simulink model "FixedWingPathDynamics"  (R2021b)
settings: Solver=VariableStepAuto  StartTime=0.0  StopTime=210  RelTol=1e-3
InitFcn:
  | FidelityStage = 2;
model workspace (MAT data in the model file):
  airspeedVal = 12.0293777094
  headingAngles : timeseries (value not decoded)
  lastWaypointInstance = [-187.583573788; -374.036820677; -81.0768]
  lookaheadPoint : timeseries (value not decoded)
  waypointData = [-39.8122089943 -39.8116872817 -39.8111647517 -39.8106414064 -39.8101172475 -39.809592277 -39.8090664968 -39.8085399087 -39.8080125146 -39.8074843164 -39.80695542 -39.8064258792 ... (1797 elements, 599x3)]
undefined symbols (not defined in the file): aircraftTmax, initialThrottle, midFidelityUAV, trimT
libraries: aerolibconvert2 x1, uavalgslib x1
(part 2 of 2)

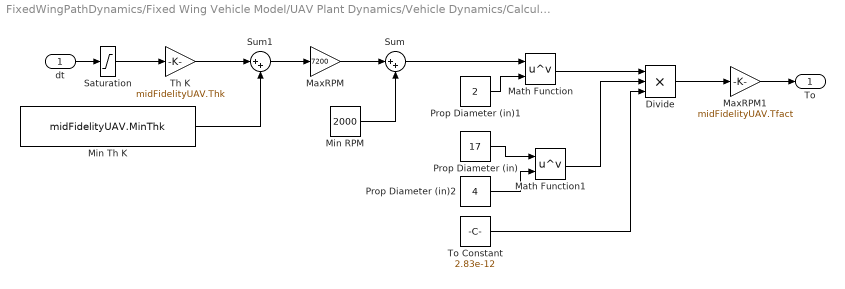
== system FixedWingPathDynamics/Fixed Wing Vehicle Model/UAV Plant Dynamics/Vehicle Dynamics/Calculate Forces/Thrust model/Advanced/Get To ==
  dt : Inport
  Divide : Product  Inputs=3
  Math Function : Math  Operator=pow  SignedPower=on  SaturateOnIntegerOverflow=on
  Math Function1 : Math  Operator=pow  SignedPower=on  SaturateOnIntegerOverflow=on
  MaxRPM : Gain  Gain=7200  SaturateOnIntegerOverflow=on  OutDataTypeStr=Inherit: Same as input  ParamDataTypeStr=Inherit: Same as input
      settings: AttributesFormatString=%<Gain>
  MaxRPM1 : Gain  Gain=midFidelityUAV.Tfact  SaturateOnIntegerOverflow=on  OutDataTypeStr=Inherit: Same as input  ParamDataTypeStr=Inherit: Same as input
      settings: AttributesFormatString=%<Gain>
  Min RPM : Constant  Value=2000
      settings: AttributesFormatString=%<Value>
  Min Th K : Constant  Value=midFidelityUAV.MinThk
      settings: AttributesFormatString=%<Value>
  Prop Diameter (in) : Constant  Value=17
      settings: AttributesFormatString=%<Value>
  Prop Diameter (in)1 : Constant  Value=2
      settings: AttributesFormatString=%<Value>
  Prop Diameter (in)2 : Constant  Value=4
      settings: AttributesFormatString=%<Value>
  Saturation : Saturate  UpperLimit=1.0  LowerLimit=0
      settings: AttributesFormatString="[%<LowerLimit>  %<UpperLimit>]"
  Sum : Sum  Inputs=|++
  Sum1 : Sum  Inputs=|++
  Th K : Gain  Gain=midFidelityUAV.Thk  SaturateOnIntegerOverflow=on  OutDataTypeStr=Inherit: Same as input  ParamDataTypeStr=Inherit: Same as input
      settings: AttributesFormatString=%<Gain>
  To Constant : Constant  Value=2.83e-12
      settings: AttributesFormatString=%<Value>
  To : Outport  VectorParamsAs1DForOutWhenUnconnected=off
  wires:
  Saturation/1 -> Th K/1
  Prop Diameter (in)1/1 -> Math Function/2
  Prop Diameter (in)2/1 -> Math Function1/2
  Prop Diameter (in)/1 -> Math Function1/1
  Math Function/1 -> Divide/1
  Math Function1/1 -> Divide/2
  To Constant/1 -> Divide/3
  Divide/1 -> MaxRPM1/1
  MaxRPM1/1 -> To/1
  Sum/1 -> Math Function/1
  Min RPM/1 -> Sum/2
  MaxRPM/1 -> Sum/1
  Th K/1 -> Sum1/1
  dt/1 -> Saturation/1
  Sum1/1 -> MaxRPM/1
  Min Th K/1 -> Sum1/2

== matlab function FixedWingPathDynamics/Heading to Bank Angle/MATLAB Function ==
  data: AirSpeed input; RollAngle output; HeadingAngle input; FlightPathAngle input; TargetHeading input; WindNorth input; WindEast input; WindDown input; Gravity input; PHeadingAngle input
function RollAngle = fcn(AirSpeed, HeadingAngle, FlightPathAngle, TargetHeading, ...
    WindNorth, WindEast, WindDown, Gravity, PHeadingAngle)

YawAngle = HeadingAngle - asin((1/AirSpeed)*[WindNorth, WindEast]*[-sin(HeadingAngle); cos(HeadingAngle)]);
b = [cos(HeadingAngle)*cos(FlightPathAngle), sin(HeadingAngle)*cos(FlightPathAngle), -sin(FlightPathAngle)]*[WindNorth; WindEast; WindDown];
c = [WindNorth, WindEast, WindDown]*[WindNorth; WindEast; WindDown]- AirSpeed^2;
Vg = -b+sqrt(b^2-c);

RollAngle = atan2(PHeadingAngle*angdiff(HeadingAngle,TargetHeading)*Vg,Gravity*cos(HeadingAngle-YawAngle));

end

== matlab function FixedWingPathDynamics/Stop Sim/MATLAB Function ==
  data: last_waypoint input; lap_val input; distance output
function distance = fcn( last_waypoint, lap_val)

  x_uav= lap_val(1);
  y_uav = lap_val(2);
  z_uav = lap_val(3);

  x_waypoint = last_waypoint(1);
  y_waypoint = last_waypoint(2);
  z_waypoint = last_waypoint(3);

  distance = sqrt((x_uav - x_waypoint)^2 + (y_uav - y_waypoint)^2 + (z_uav - z_waypoint)^2);
  if distance < 5
      disp(distance)
  end
